simulink model "test1"  (R2017b)
settings: Solver=VariableStepAuto  StartTime=0.0  StopTime=50  RelTol=1e-3
settings Model: Creator=Administrator  LastModifiedBy=Administrator

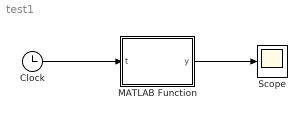
== system test1 ==
  Clock : Clock
  MATLAB Function : MATLAB Function  TreatAsAtomicUnit=on
  Scope : Scope
  wires:
  Clock/1 -> MATLAB Function/1(t)
  MATLAB Function/1(y) -> Scope/1

== matlab function test1/MATLAB Function ==
  data: t input; y output
function y = circle1(t)
x=0.01*t;
rx1=0;ry1=0.04;r1=0.04; 
rx2=0.05*sqrt(2);ry2=0.04-0.05*sqrt(2);r2=0.06;
rx3=(rx2+0.07);ry3=ry2+0.07*sqrt(3);r3=0.08;
rx4=(rx3+0.085);ry4=ry3-0.085*sqrt(3);r4=0.09;
rx5=(rx4+0.06);ry5=ry4+0.06*sqrt(3);r5=0.03;

if t<(2*sqrt(2))
y=ry1-(r1^2-(x-rx1)^2)^0.5;

elseif (2*sqrt(2))<t && t<(5*sqrt(2)+3)
y=ry2+abs((r2^2-(x-rx2)^2))^0.5;

elseif (5*sqrt(2)+3)<t && t<(5*sqrt(2)+11)
y=ry3-abs((r3^2-(x-rx3)^2))^0.5;

elseif t>5*sqrt(2)+11 && t<5*sqrt(2)+20
y=ry4+abs((r4^2-(x-rx4)^2))^0.5;

elseif (5*sqrt(2)+20<t) && (t<(5*sqrt(2)+21.5))
y=ry5-abs((r5^2-(x-rx5)^2))^0.5;
   
else
    y=ry5-0.018*sqrt(3);

end
